simulink model "EGH"  (R2025a)
settings: Solver=VariableStepAuto  StartTime=0.0  StopTime=20e-3  MaxStep=0.5e-3/50  RelTol=1e-3
libraries: MSZSZ_MK x3
settings Model: Creator=Szalay  LastModifiedBy=Szalay

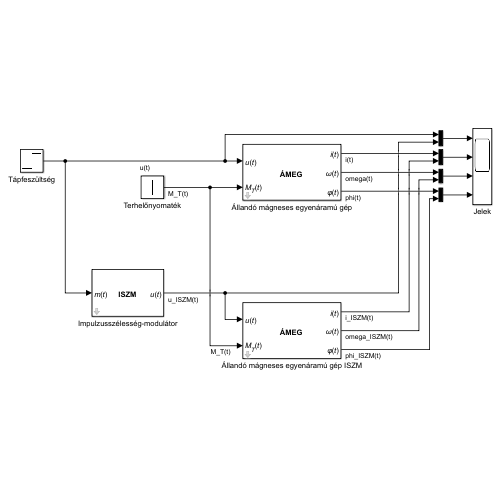
[thumbnail: Simulink's stored preview of the top-level diagram]
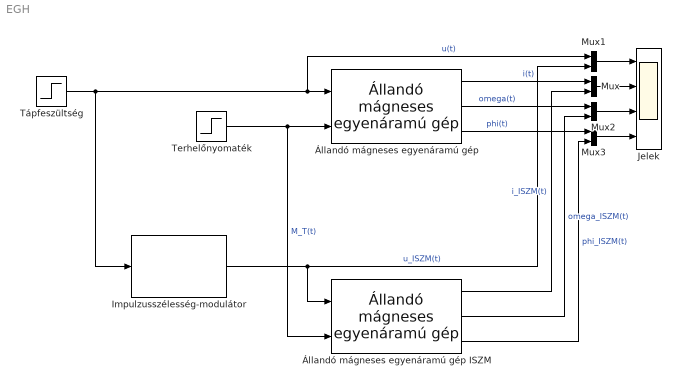
== system EGH ==
  Impulzusszélesség-modulátor : MSZSZ_MK/Impulzusszélesség-modulátor  U_T=18  f_ISZM=20000  T_D=1e-6
  Jelek : Scope  NumInputPorts=4
      settings: ActiveDisplayString=4  ActiveDisplayYMinimum=-0.40295544051422622  ActiveDisplayYMaximum=3.6264679807362539
  Mux{,1..3} (4 alike) : Mux  Inputs=2
  Terhelőnyomaték : Step  Time=10e-3  After=200e-3  SampleTime=0
  Tápfeszültség : Step  Time=1e-3  After=9  SampleTime=0
  Állandó mágneses egyenáramú gép : MSZSZ_MK/Állandó mágneses egyenáramú gép  R=212e-3  L=77e-6  k_T=23.4e-3  k_E=23.4e-3  J=102e-7  B=5.4932e-6  i_0=0  omega_0=0  phi_0=0
  Állandó mágneses egyenáramú gép ISZM : MSZSZ_MK/Állandó mágneses egyenáramú gép  R=212e-3  L=77e-6  k_T=23.4e-3  k_E=23.4e-3  J=102e-7  B=5.4932e-6  i_0=0  omega_0=0  phi_0=0
  wires:
  Állandó mágneses egyenáramú gép/1 -> Mux/1  "i(t)"
  Állandó mágneses egyenáramú gép/2 -> Mux2/1  "omega(t)"
  Állandó mágneses egyenáramú gép/3 -> Mux3/1  "phi(t)"
  Terhelőnyomaték/1 -> Állandó mágneses egyenáramú gép ISZM/2, Állandó mágneses egyenáramú gép/2  "M_T(t)"
  Állandó mágneses egyenáramú gép ISZM/3 -> Mux3/2  "phi_ISZM(t)"
  Állandó mágneses egyenáramú gép ISZM/2 -> Mux2/2  "omega_ISZM(t)"
  Állandó mágneses egyenáramú gép ISZM/1 -> Mux/2  "i_ISZM(t)"
  Tápfeszültség/1 -> Mux1/1, Állandó mágneses egyenáramú gép/1, Impulzusszélesség-modulátor/1  "u(t)"
  Impulzusszélesség-modulátor/1 -> Állandó mágneses egyenáramú gép ISZM/1, Mux1/2  "u_ISZM(t)"
  Mux1/1 -> Jelek/1
  Mux/1 -> Jelek/2
  Mux2/1 -> Jelek/3
  Mux3/1 -> Jelek/4
